simulink model "static_arc"  (R2025b)
settings: Solver=VariableStepAuto  StartTime=0.0  StopTime=10.0  RelTol=1e-3
model workspace (MAT data in the model file):
  K1 = 221320
  K2 = 0.00072
  U_PhaseRMS = 243
  Xd = 0.003
  lambda = 2
  rd = 0.0004
settings Model: Creator=LYG  LastModifiedBy=LYG

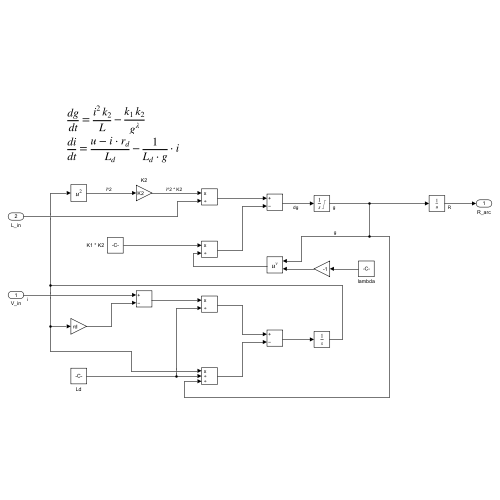
[thumbnail: Simulink's stored preview of the top-level diagram]
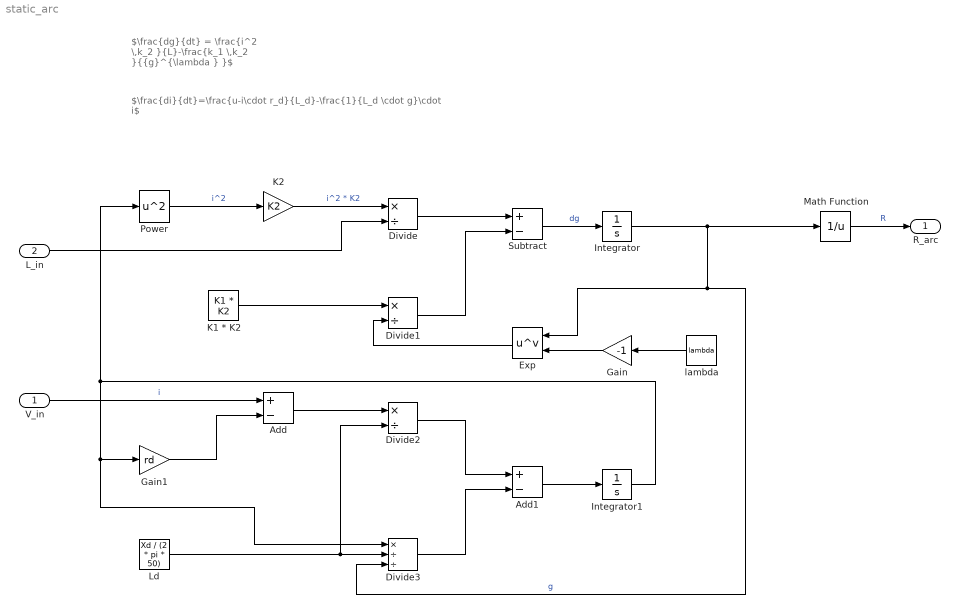
== system static_arc ==
  note: $\frac{di}{dt}=\frac{u-i\cdot r_d}{L_d}-\frac{1}{L_d \cdot g}\cdot i$
  note: $\frac{dg}{dt} = \frac{i^2 \,k_2 }{L}-\frac{k_1 \,k_2 }{{g}^{\lambda } }$
  V_in : Inport
  L_in : Inport  Port=2
  Add : Sum  Inputs=+-
  Add1 : Sum  Inputs=+-
  Divide : Product  Inputs=*/
  Divide1 : Product  Inputs=*/
  Divide2 : Product  Inputs=*/
  Divide3 : Product  Inputs=*//
  Exp : Math  Operator=pow
  Gain : Gain  Gain=-1
  Gain1 : Gain  Gain=rd
  Integrator : Integrator  InitialCondition=50  LimitOutput=on  UpperSaturationLimit=1e3  LowerSaturationLimit=1e-3
  Integrator1 : Integrator
  K1 * K2 : Constant  Value=K1 * K2
  K2 : Gain  Gain=K2
  Ld : Constant  Value=Xd / (2 * pi * 50)
  Math Function : Math  Operator=reciprocal
  Power : Math  Operator=square
  Subtract : Sum  Inputs=+-
  lambda : Constant  Value=lambda
  R_arc : Outport
  wires:
  Gain/1 -> Exp/2
  Divide1/1 -> Subtract/2
  Subtract/1 -> Integrator/1  "dg"
  Math Function/1 -> R_arc/1  "R"
  Divide/1 -> Subtract/1
  Power/1 -> K2/1  "i^2"
  lambda/1 -> Gain/1
  K1 * K2/1 -> Divide1/1
  K2/1 -> Divide/1  "i^2 * K2"
  Integrator/1 -> Math Function/1, Exp/1, Divide3/3  "g"
  Exp/1 -> Divide1/2
  L_in/1 -> Divide/2
  V_in/1 -> Add/1  "i"
  Gain1/1 -> Add/2
  Add/1 -> Divide2/1
  Ld/1 -> Divide2/2, Divide3/2
  Divide2/1 -> Add1/1
  Divide3/1 -> Add1/2
  Add1/1 -> Integrator1/1
  Integrator1/1 -> Power/1, Divide3/1, Gain1/1
